simulink model "prblm1"  (R2020b)
settings: Solver=VariableStepAuto  StartTime=0.0  StopTime=10.0  RelTol=1e-3
settings Model: Creator=Shree  LastModifiedBy=Shree

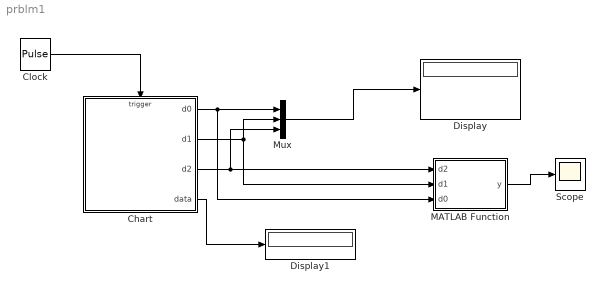
== system prblm1 ==
  Chart : Stateflow chart  TreatAsAtomicUnit=on
  Clock : DiscretePulseGenerator  PulseType=Time based  Period=0.5  PulseWidth=5
  Display : Display
  Display1 : Display
  MATLAB Function : MATLAB Function  TreatAsAtomicUnit=on
  Mux : Mux  Inputs=3
  Scope : Scope
  wires:
  Chart/4(data) -> Display1/1
  Clock/1 -> Chart/Trigger
  Mux/1 -> Display/1
  Chart/1(d0) -> Mux/1, MATLAB Function/3(d0)
  Chart/2(d1) -> Mux/2, MATLAB Function/2(d1)
  MATLAB Function/1(y) -> Scope/1
  Chart/3(d2) -> MATLAB Function/1(d2), Mux/3

== matlab function prblm1/MATLAB Function ==
  data: d2 input; y output; d1 input; d0 input
function y= fcn(d2,d1,d0)
if(d2==0 && d1==0 && d0==0)
    y=0;
elseif(d2==0 && d1==0 && d0==1)
    y=1;
elseif(d2==0 && d1==1 && d0==0)
    y=2;
elseif(d2==0 && d1==1 && d0==1)
    y=3;
elseif(d2==1 && d1==0 && d0==0)
    y=4;
else
    y=0;
    
end

== stateflow chart prblm1/Chart ==
  state ConversionState [parallel]
    during:
    data2=d2;
    data1=d1;
    data0=d0;
    r=0;
    check(data2,data1,data0);
    settings: executionOrder=4
  state digit0 [parallel]
    settings: executionOrder=1
    state zero
      en:
      d0=0;
    state one
      en:
      d0=1
    digit0.one -> digit0.zero [order 2] : [r==1]
    (default) -> digit0.zero
    digit0.one -> digit0.zero [order 1] : pulse{send(inc1);}
    digit0.zero -> digit0.one : pulse
  note: 000-0
      | 001-1
      | 010-2
      | 011-3
      | 100-4
      | 101-5
      | 110-6
      | 111-7
  state check(d02,d01,d00) [function]
    (default) -> (junction 123) : % Conversion to Decimal
    (junction 123) -> (junction 128) [order 1] : [d02==0 && d01==0 && d00==0]
    (junction 123) -> (junction 124) [order 2]
    (junction 128) -> (junction 150) : {data=0;
        | r=0;}
    (junction 124) -> (junction 126) [order 1] : [d02==0 && d01==0 && d00==1]
    (junction 124) -> (junction 127) [order 2]
    (junction 126) -> (junction 137) : {data=1;
        | r=0;}
    (junction 127) -> (junction 125) [order 1] : [d02==0 && d01==1 && d00==0]
    (junction 127) -> (junction 129) [order 2]
    (junction 125) -> (junction 131) : {data=2;
        | r=0;}
    (junction 129) -> (junction 134) [order 1] : [d02==0 && d01==1 && d00==1]
    (junction 129) -> (junction 187) [order 2]
    (junction 134) -> (junction 133) : {data=3;
        | r=0;}
    (junction 187) -> (junction 132) [order 1] : [d02==1 && d01==0 && d00==0]
    (junction 187) -> (junction 130) [order 2]
    (junction 132) -> (junction 136) : {data=4;
        | r=0;}
    (junction 136) -> (junction 130)
    (junction 133) -> (junction 136)
    (junction 131) -> (junction 133)
    (junction 137) -> (junction 131)
    (junction 150) -> (junction 137)
    (junction 130) -> (junction 143)
  state digit1 [parallel]
    settings: executionOrder=2
    state zero
      en:
      d1=0;
    state one
      en:
      d1=1;
    (default) -> digit1.zero
    digit1.one -> digit1.zero : inc1{send(inc2);}
    digit1.zero -> digit1.one : inc1
  state digit2 [parallel]
    settings: executionOrder=3
    state zero
      en:
      d2=0;
    state one
      en:
      d2=1;
    (default) -> digit2.zero
    digit2.one -> digit2.zero : inc2
    digit2.zero -> digit2.one : inc2
  (default) -> digit0
  data: d02 function_input; d01 function_input; d00 function_input; d0 output; d1 output; d2 output; data output; data0 local; data1 local; data2 local; r local; re local; i local
  events: pulse input RISING_EDGE_EVENT; inc1 local FUNCTION_CALL_EVENT; inc2 local FUNCTION_CALL_EVENT; reset local EITHER_EDGE_EVENT
